simulink library "relay_housing_lib"  (Simulink 8.1)
settings: Solver=ode45  StartTime=0.0  StopTime=10.0  RelTol=1e-3
values from neighbouring files (symbols this model uses):
  Ts = 100E-6    (= 0.0001)    [BANSHEE_init.m]
undefined symbols (not defined in the file or in its folder): F1, F2, F3, generic_ethernet_cb
libraries: relay_modbus_lib x42, rtio_generic_modbus x42, rtlab x5, udp_powerfactor_lib x3, PQFV_lib x3, opal_lib x1, LoadProfiles_lib x1
(part 2 of 2)

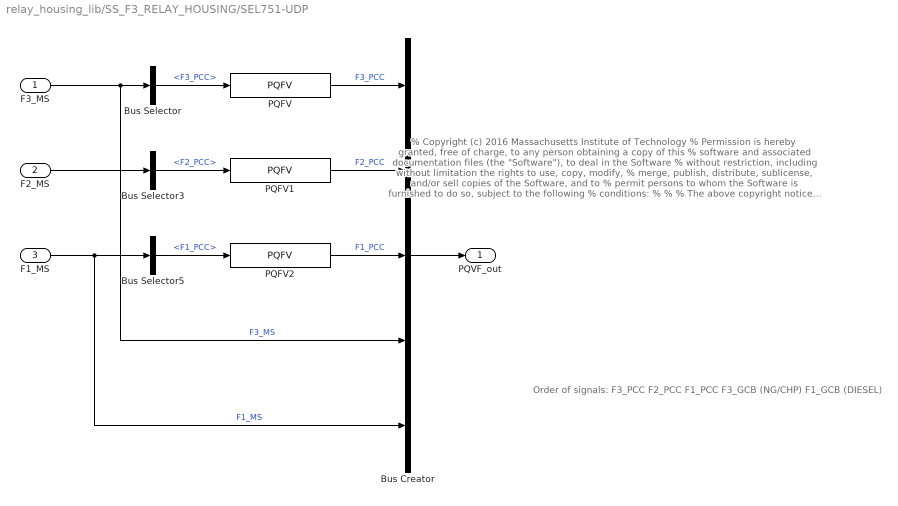
== system relay_housing_lib/SS_F3_RELAY_HOUSING/SEL751-UDP ==
  note: % Copyright (c) 2016 Massachusetts Institute of Technology
      | % Permission is hereby granted, free of charge, to any person obtaining a copy of this
      | % software and associated documentation files (the "Software"), to deal in the Software
      | % without restriction, including without limitation the rights to use, copy, modify,
      | % merge, publish, distribute, sublicense, and/or sell copies of the Software, and to
      | % permit persons to whom the Software is furnished to do so, subject to the following
      | % conditions:
      | %
      | %
      | % The above copyright notice and this permission notice shall be included in
      | % all copies or substantial portions of the Software.
      | %
      | % THE SOFTWARE IS PROVIDED "AS IS", WITHOUT WARRANTY OF ANY KIND, EXPRESS OR IMPLIED,
      | % INCLUDING BUT NOT LIMITED TO THE WARRANTIES OF MERCHANTABILITY, FITNESS FOR A
      | % PARTICULAR PURPOSE AND NONINFRINGEMENT. IN NO EVENT SHALL THE AUTHORS OR COPYRIGHT
      | % HOLDERS BE LIABLE FOR ANY CLAIM, DAMAGES OR OTHER LIABILITY, WHETHER IN AN ACTION
      | % OF CONTRACT, TORT OR OTHERWISE, ARISING FROM, OUT OF OR IN CONNECTION WITH THE
      | % SOFTWARE OR THE USE OR OTHER DEALINGS IN THE SOFTWARE.
      | %
      | %
      | %%
  note: Order of signals:
      | F3_PCC
      | F2_PCC
      | F1_PCC
      | F3_GCB (NG/CHP)
      | F1_GCB (DIESEL)
  F3_MS : Inport
  F2_MS : Inport  Port=2
  F1_MS : Inport  Port=3
  Bus Creator : BusCreator  Inputs=5
  Bus Selector : BusSelector  OutputSignals=CB_DATA.F3_PCC
  Bus Selector3 : BusSelector  OutputSignals=CB_DATA.F2_PCC
  Bus Selector5 : BusSelector  OutputSignals=CB_DATA.F1_PCC
  PQFV : PQFV_lib/PQFV  VRMSLL=13800
  PQFV1 : PQFV_lib/PQFV  VRMSLL=13800
  PQFV2 : PQFV_lib/PQFV  VRMSLL=13800
  PQVF_out : Outport
  wires:
  Bus Creator/1 -> PQVF_out/1
  F1_MS/1 -> Bus Selector5/1, Bus Creator/5  "F1_MS"
  F3_MS/1 -> Bus Selector/1, Bus Creator/4  "F3_MS"
  PQFV2/1 -> Bus Creator/3  "F1_PCC"
  PQFV/1 -> Bus Creator/1  "F3_PCC"
  PQFV1/1 -> Bus Creator/2  "F2_PCC"
  Bus Selector5/1 -> PQFV2/1  "<F1_PCC>"
  F2_MS/1 -> Bus Selector3/1
  Bus Selector3/1 -> PQFV1/1  "<F2_PCC>"
  Bus Selector/1 -> PQFV/1  "<F3_PCC>"

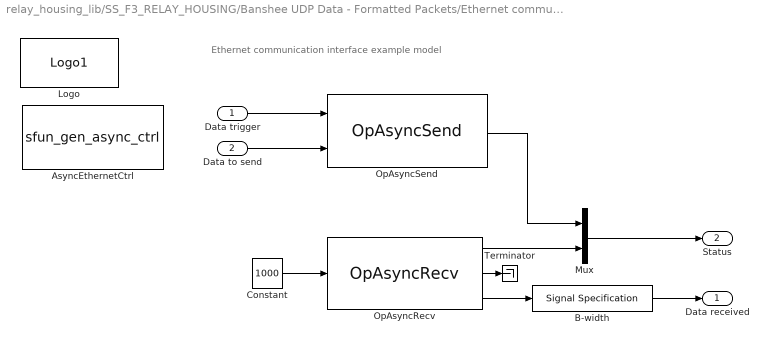
== system relay_housing_lib/SS_F3_RELAY_HOUSING/Banshee UDP Data - Formatted Packets/Ethernet communication interface ==
  note: Ethernet communication interface example model
  Data trigger : Inport
  Data to send : Inport  Port=2
  AsyncEthernetCtrl : S-Function  InitFcn=generic_ethernet_cb('initfcn');  FunctionName=sfun_gen_async_ctrl  Parameters=ctrl_id, nbr_to_remote_endpoint, type_to_remote_endpoint,nbr_from_remote_endpoint,type_from_remote_endpoint,protocol,tcp_mode, port, offset_to_remote_endpoint,offset_from_remote_endpoint,swap_tx,swap_rx,0,nic_name,remote_ip,'','','','','','','','','','',exe_name,0  EnableBusSupport=off  mask(AsyncEthernetCtrl){ctrl_id=1, nbr_to_remote_endpoint=332, type_to_remote_endpoint=INT32, offset_to_remote_endpoint=0, nbr_from_remote_endpoint=4, type_from_remote_endpoint=DOUBLE, offset_from_remote_endpoint=0, nic_name=eth0, protocol=UDP, tcp_mode=Server, port=7200, remote_ip=255.255.255.255, exe_name=AsyncEthernet, swap_tx=off, swap_rx=off}
      mask prompts: ctrl_id "Controller ID"; nbr_to_remote_endpoint "Number of data to send"; type_to_remote_endpoint "Type of data to send"; offset_to_remote_endpoint "Byte offset of transmission buffer"; nbr_from_remote_endpoint "Number of data expected to be received"; type_from_remote_endpoint "Type of data expected to be received"; offset_from_remote_endpoint "Byte offset of reception buffer"; nic_name "Network interface name"; tcp_mode "TCP mode"; remote_ip "Remote IP address"; exe_name "Name of the executable"; swap_tx "Swap data endianness before transmission"; swap_rx "Swap data endianness after reception"
      mask help: Generic asynchronous process configuration block
      mask Help: eval('rtlab_help(''opasyncgenctrl'');');
      mask TypeOptions type_to_remote_endpoint: UINT8 | INT8 | UINT16 | INT16 | UINT32 | INT32 | FLOAT | DOUBLE
      mask TypeOptions type_from_remote_endpoint: UINT8 | INT8 | UINT16 | INT16 | UINT32 | INT32 | FLOAT | DOUBLE
      mask TypeOptions protocol: UDP | TCP
      mask TypeOptions tcp_mode: Client | Server
      mask Display: disp(sprintf('\nEthernet communication \ninterface controller\n'))
  B-width : SignalSpecification  Dimensions=nbr_from_remote_endpoint
  Constant : Constant  Value=1000
  Logo : opal_lib/Logo1  vide=[]
  Mux : Mux  Inputs=2
  OpAsyncRecv : rtlab/Communication/Asynchronous/OpAsyncRecv  ctl_id=ctrl_id  recv_id=ctrl_id  enable_param=off  fp1=1  fp2=2  fp3=3  fp4=4  fp5=5  sp1=string1  sp2=string2  sp3=string3  sp4=string4  sp5=string5
  OpAsyncSend : rtlab/Communication/Asynchronous/OpAsyncSend  ctl_id=ctrl_id  send_id=ctrl_id  mode=DONT_NEED_REPLY  enable_param=off  fp1=1  fp2=2  fp3=3  fp4=4  fp5=5  sp1=string1  sp2=string2  sp3=string3  sp4=string4  sp5=string5
  Terminator : Terminator
  Data received : Outport
  Status : Outport  Port=2
  wires:
  B-width/1 -> Data received/1
  OpAsyncRecv/3 -> B-width/1
  OpAsyncRecv/2 -> Terminator/1
  Constant/1 -> OpAsyncRecv/1
  Mux/1 -> Status/1
  OpAsyncRecv/1 -> Mux/2
  OpAsyncSend/1 -> Mux/1
  Data trigger/1 -> OpAsyncSend/1
  Data to send/1 -> OpAsyncSend/2

== matlab function SS_F3_RELAY_HOUSING/Banshee UDP Data - Formatted Packets/Cast uint16 ==
  data: u input double; y output double
function y = fcn(u)
%#codegen

x = double(typecast(uint32(u),'uint16'));
y = x(1); % low bits
